simulink model "Lab2_Demo"  (R2020a)
settings: Solver=FixedStepAuto  StartTime=0.0  StopTime=10.0  FixedStep=1e-3  RelTol=1e-3  EnableMultiTasking=on
undefined symbols (not defined in the file): pip
libraries: frdmk64flib x2
settings Model: ExtModeTrigDuration=5  Creator=forre  LastModifiedBy=forre
settings OptimizationCC: EnhancedBackFolding=on  PassReuseOutputArgsAs=Individual arguments  ZeroExternalMemoryAtStartup=off  ZeroInternalMemoryAtStartup=off  MaxStackSize=64  OptimizeBlockOrder=speed  DifferentSizesBufferReuse=on  OptimizationCustomize=off  EfficientTunableParamExpr=on
settings DebuggingCC: ParameterTunabilityLossMsg=error
settings HardwareCC: ProdBitPerPointer=32  ProdBitPerSizeT=32  ProdBitPerPtrDiffT=32  ProdLargestAtomicInteger=Long  ProdLargestAtomicFloat=Double  ProdWordSize=32  ProdHWDeviceType=ARM Compatible->ARM Cortex
settings SFSimCC: MATLABDynamicMemAlloc=off
settings RTWCC: SystemTargetFile=ert.tlc  HardwareBoard=NXP FRDM-K64F  TemplateMakefile=ert_default_tmf  Toolchain=GNU Tools for ARM Embedded Processors
settings CodeAppCC: ForceParamTrailComments=on  IgnoreCustomStorageClasses=off  OperatorAnnotations=on  SimulinkDataObjDesc=on  SFDataObjDesc=on  InsertBlockDesc=on

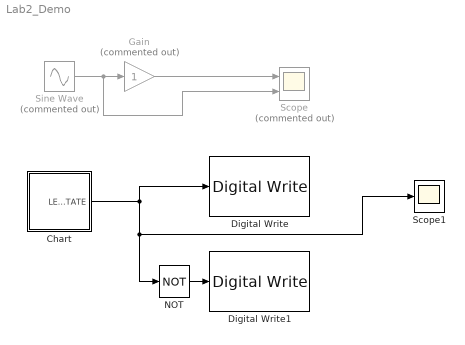
== system Lab2_Demo ==
  Chart : Stateflow chart  TreatAsAtomicUnit=on
  Digital Write : frdmk64flib/Digital Write  Whichpin=RED_LED
  Digital Write1 : frdmk64flib/Digital Write  Whichpin=GREEN_LED
  Gain : Gain  Commented=on
  NOT : Logic  Operator=NOT  IconShape=distinctive  AllPortsSameDT=off  OutDataTypeStr=boolean
  Scope : Scope  Commented=on  NumInputPorts=2
  Scope1 : Scope
  Sine Wave : Sin  Commented=on  Amplitude=2  Frequency=pip  Phase=pi/2  SampleTime=0
  wires:
  Gain/1 -> Scope/1
  Sine Wave/1 -> Scope/2, Gain/1
  Chart/1(LED_STATE) -> Scope1/1, NOT/1, Digital Write/1
  NOT/1 -> Digital Write1/1

== stateflow chart Lab2_Demo/Chart ==
  state LED_OFF
    entry:
    LED_STATE = false;
  state LED_ON
    entry:
    LED_STATE = true;
  (default) -> LED_OFF
  LED_OFF -> LED_ON : after(1000,msec)
  LED_ON -> LED_OFF : after(1000,msec)
  data: LED_STATE output boolean
